simulink model "Mdl_TurnHazard"  (R2024b)
settings: Solver=FixedStepDiscrete  StartTime=0.0  StopTime=10.0  FixedStep=0.1  RelTol=1e-3  EnableMultiTasking=on
values from neighbouring files (symbols this model uses):
  cTH_ONE = mpt.Parameter    [Mdl_TurnHazard_DD.m]
  cTH_THREE = mpt.Parameter    [Mdl_TurnHazard_DD.m]
  cTH_TWO = mpt.Parameter    [Mdl_TurnHazard_DD.m]
undefined symbols (not defined in the file or in its folder): CLUSTER_INACTIVE, eSIGNAL_OK, eTurn_Indicator_ControlIn, tRxSignalId_type_instance, tRxSignalStatus_type_instance, TT_TURN_OFF, TT_TURN_ON, TurnBlink, TurnOff
libraries: simulink x1
settings Model: Creator=aelango6  LastModifiedBy=aelango6
settings DataIOCC: SaveOutput=off
settings OptimizationCC: DefaultParameterBehavior=Inlined  EnhancedBackFolding=on  PassReuseOutputArgsAs=Individual arguments  ZeroExternalMemoryAtStartup=off  ZeroInternalMemoryAtStartup=off  MaxStackSize=750  OptimizeBlockOrder=speed  DifferentSizesBufferReuse=on  OptimizationCustomize=off  EfficientTunableParamExpr=on
settings DebuggingCC: ParameterTunabilityLossMsg=error
settings SFSimCC: MATLABDynamicMemAlloc=off
settings RTWCC: Description=AUTOSAR  SystemTargetFile=autosar.tlc  GenCodeOnly=on  TemplateMakefile=ert_default_tmf  PortableWordSizes=on  DataTypeReplacement=CDataTypesFixedWidth
settings CodeAppCC: ForceParamTrailComments=on  IgnoreCustomStorageClasses=off  OperatorAnnotations=on  SimulinkDataObjDesc=on  SFDataObjDesc=on  InsertBlockDesc=on
settings STFCustomTargetCC: TargetLangStandard=C99 (ISO)  MultiwordLength=256  ParMdlRefBuildCompliant=on  CompOptLevelCompliant=on  IncludeMdlTerminateFcn=off  CombineOutputUpdateFcns=on  SuppressErrorStatus=on  ERTCustomFileBanners=on  SupportNonFinite=off  SupportComplex=off  SupportContinuousTime=off  SupportNonInlinedSFcns=off  RemoveResetFunc=on  ParenthesesLevel=Maximum  CastingMode=Standards  MATLABClassNameForMDSCustomization=Simulink.SoftwareTarget.ERTCustomization  AutosarCompliant=on  UseToolchainInfoCompliant=on  LookupTableObjectStructAxisOrder=2,1,3,4,...  LUTObjectStructOrderEvenSpacing=Size,Table,Breakpoints  SystemTargetFile=autosar.tlc
settings ERTTargetCC: TargetLangStandard=C99 (ISO)  ConcurrentExecutionCompliant=off  IncludeMdlTerminateFcn=off  SuppressErrorStatus=on  SupportNonFinite=off  SupportComplex=off  ParenthesesLevel=Maximum  CastingMode=Standards  ModelStepFunctionPrototypeControlCompliant=off  CPPClassGenCompliant=off  AutosarCompliant=on  LookupTableObjectStructAxisOrder=2,1,3,4,...  LUTObjectStructOrderEvenSpacing=Size,Table,Breakpoints  ERTCustomFileTemplate=example_file_process.tlc  ERTFilePackagingFormat=CompactWithDataFile  BooleanTrueId=TRUE  BooleanFalseId=FALSE

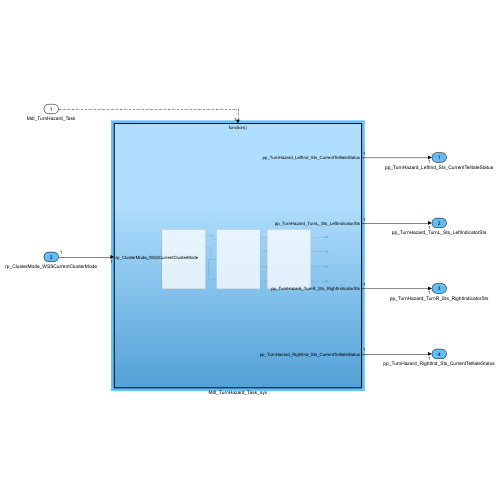
[thumbnail: Simulink's stored preview of the top-level diagram]
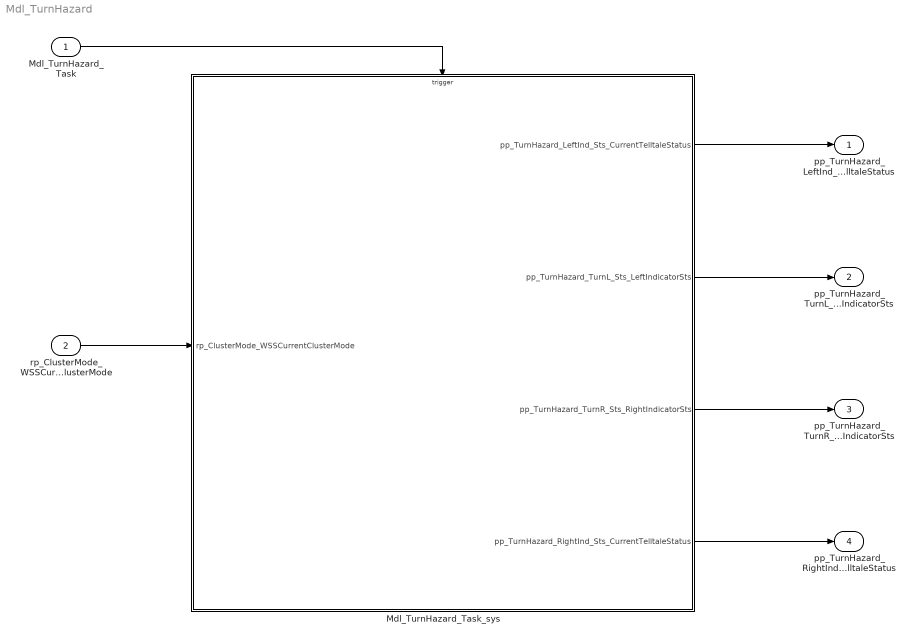
== system Mdl_TurnHazard ==
  Mdl_TurnHazard_Task : Inport  SampleTime=0.1  OutputFunctionCall=on
  rp_ClusterMode_WSSCurrentClusterMode : Inport  Port=2  OutDataTypeStr=ClusterModes  PortDimensions=1
  Mdl_TurnHazard_Task_sys : Subsystem  TreatAsAtomicUnit=on
  pp_TurnHazard_LeftInd_Sts_CurrentTelltaleStatus : Outport  OutDataTypeStr=TT_OP_STATES
  pp_TurnHazard_TurnL_Sts_LeftIndicatorSts : Outport  Port=2  OutDataTypeStr=TurnStates
  pp_TurnHazard_TurnR_Sts_RightIndicatorSts : Outport  Port=3  OutDataTypeStr=TurnStates
  pp_TurnHazard_RightInd_Sts_CurrentTelltaleStatus : Outport  Port=4  OutDataTypeStr=TT_OP_STATES
  wires:
  Mdl_TurnHazard_Task_sys/1(pp_TurnHazard_LeftInd_Sts_CurrentTelltaleStatus) -> pp_TurnHazard_LeftInd_Sts_CurrentTelltaleStatus/1
  Mdl_TurnHazard_Task/1 -> Mdl_TurnHazard_Task_sys/Trigger
  Mdl_TurnHazard_Task_sys/3(pp_TurnHazard_TurnR_Sts_RightIndicatorSts) -> pp_TurnHazard_TurnR_Sts_RightIndicatorSts/1
  rp_ClusterMode_WSSCurrentClusterMode/1 -> Mdl_TurnHazard_Task_sys/1(rp_ClusterMode_WSSCurrentClusterMode)
  Mdl_TurnHazard_Task_sys/2(pp_TurnHazard_TurnL_Sts_LeftIndicatorSts) -> pp_TurnHazard_TurnL_Sts_LeftIndicatorSts/1
  Mdl_TurnHazard_Task_sys/4(pp_TurnHazard_RightInd_Sts_CurrentTelltaleStatus) -> pp_TurnHazard_RightInd_Sts_CurrentTelltaleStatus/1

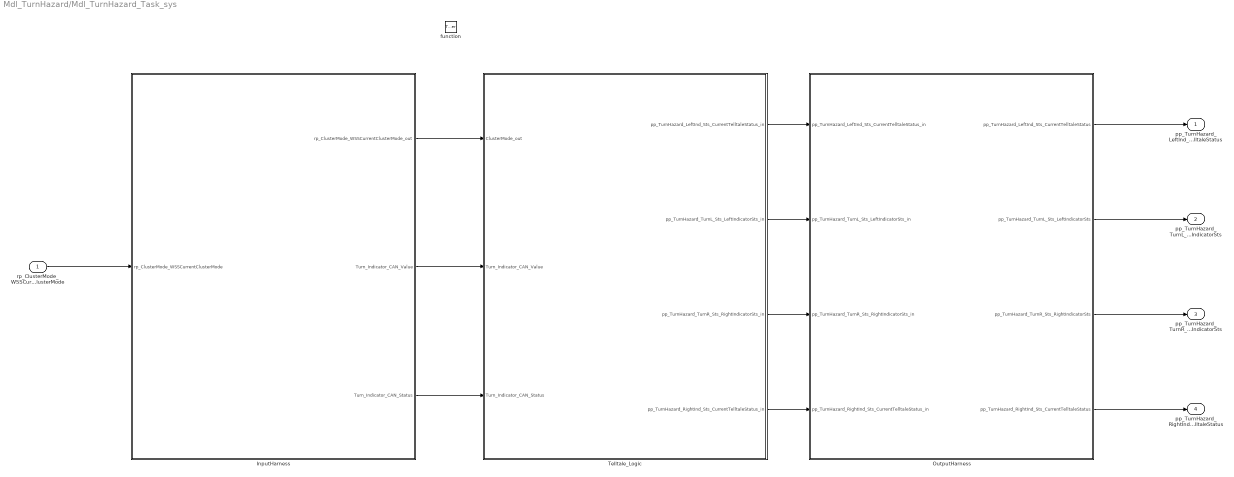
== system Mdl_TurnHazard/Mdl_TurnHazard_Task_sys ==
  rp_ClusterMode_WSSCurrentClusterMode : Inport  OutDataTypeStr=ClusterModes  PortDimensions=1
  function : TriggerPort  TriggerType=function-call  VariantControl=(inherit)  SampleTimeType=periodic  SampleTime=-1
  InputHarness : Subsystem  Variant=on
  OutputHarness : Subsystem  Variant=on
  Telltale_Logic : Subsystem  Description=|
      | Input 1 : Deboune Count
      | Input 2 : Reset Timer Status
      | Output : Timer Debounce Status
  pp_TurnHazard_LeftInd_Sts_CurrentTelltaleStatus : Outport  OutDataTypeStr=TT_OP_STATES  PortDimensions=1
  pp_TurnHazard_TurnL_Sts_LeftIndicatorSts : Outport  Port=2  OutDataTypeStr=TurnStates  PortDimensions=1
  pp_TurnHazard_TurnR_Sts_RightIndicatorSts : Outport  Port=3  OutDataTypeStr=TurnStates  PortDimensions=1
  pp_TurnHazard_RightInd_Sts_CurrentTelltaleStatus : Outport  Port=4  OutDataTypeStr=TT_OP_STATES  PortDimensions=1
  wires:
  rp_ClusterMode_WSSCurrentClusterMode/1 -> InputHarness/1(rp_ClusterMode_WSSCurrentClusterMode)
  InputHarness/1(rp_ClusterMode_WSSCurrentClusterMode_out) -> Telltale_Logic/1(ClusterMode_out)
  InputHarness/3(Turn_Indicator_CAN_Status) -> Telltale_Logic/3(Turn_Indicator_CAN_Status)
  InputHarness/2(Turn_Indicator_CAN_Value) -> Telltale_Logic/2(Turn_Indicator_CAN_Value)
  Telltale_Logic/1(pp_TurnHazard_LeftInd_Sts_CurrentTelltaleStatus_in) -> OutputHarness/1(pp_TurnHazard_LeftInd_Sts_CurrentTelltaleStatus_in)
  Telltale_Logic/2(pp_TurnHazard_TurnL_Sts_LeftIndicatorSts_in) -> OutputHarness/2(pp_TurnHazard_TurnL_Sts_LeftIndicatorSts_in)
  Telltale_Logic/3(pp_TurnHazard_TurnR_Sts_RightIndicatorSts_in) -> OutputHarness/3(pp_TurnHazard_TurnR_Sts_RightIndicatorSts_in)
  Telltale_Logic/4(pp_TurnHazard_RightInd_Sts_CurrentTelltaleStatus_in) -> OutputHarness/4(pp_TurnHazard_RightInd_Sts_CurrentTelltaleStatus_in)
  OutputHarness/1(pp_TurnHazard_LeftInd_Sts_CurrentTelltaleStatus) -> pp_TurnHazard_LeftInd_Sts_CurrentTelltaleStatus/1
  OutputHarness/2(pp_TurnHazard_TurnL_Sts_LeftIndicatorSts) -> pp_TurnHazard_TurnL_Sts_LeftIndicatorSts/1
  OutputHarness/3(pp_TurnHazard_TurnR_Sts_RightIndicatorSts) -> pp_TurnHazard_TurnR_Sts_RightIndicatorSts/1
  OutputHarness/4(pp_TurnHazard_RightInd_Sts_CurrentTelltaleStatus) -> pp_TurnHazard_RightInd_Sts_CurrentTelltaleStatus/1

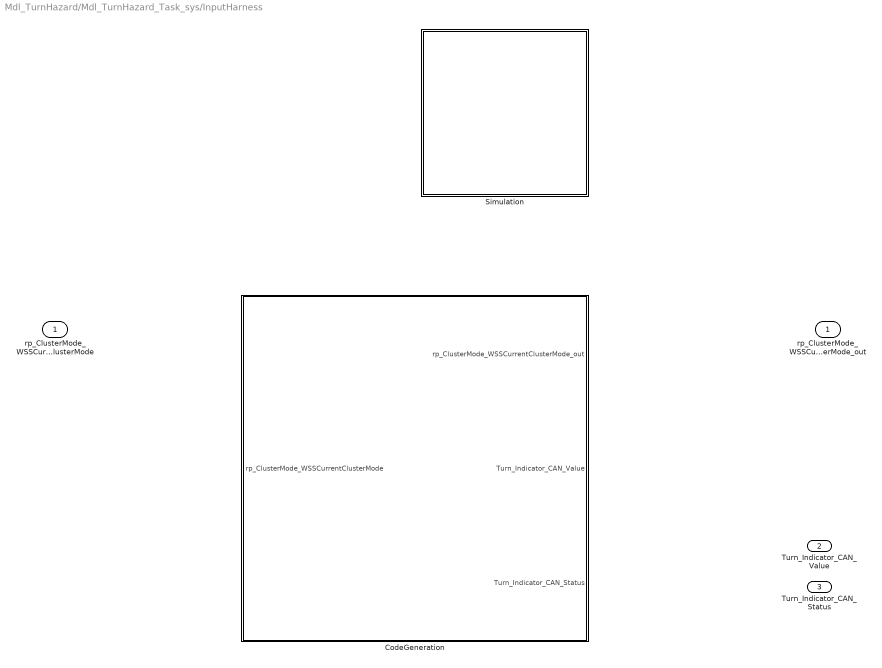
== system Mdl_TurnHazard/Mdl_TurnHazard_Task_sys/InputHarness ==
  rp_ClusterMode_WSSCurrentClusterMode : Inport  OutDataTypeStr=ClusterModes  PortDimensions=1
  CodeGeneration : Subsystem  VariantControl=CODEGENERATION
  Simulation : Subsystem  VariantControl=SIMULATION
  rp_ClusterMode_WSSCurrentClusterMode_out : Outport  OutDataTypeStr=ClusterModes  PortDimensions=1
  Turn_Indicator_CAN_Value : Outport  Port=2
  Turn_Indicator_CAN_Status : Outport  Port=3

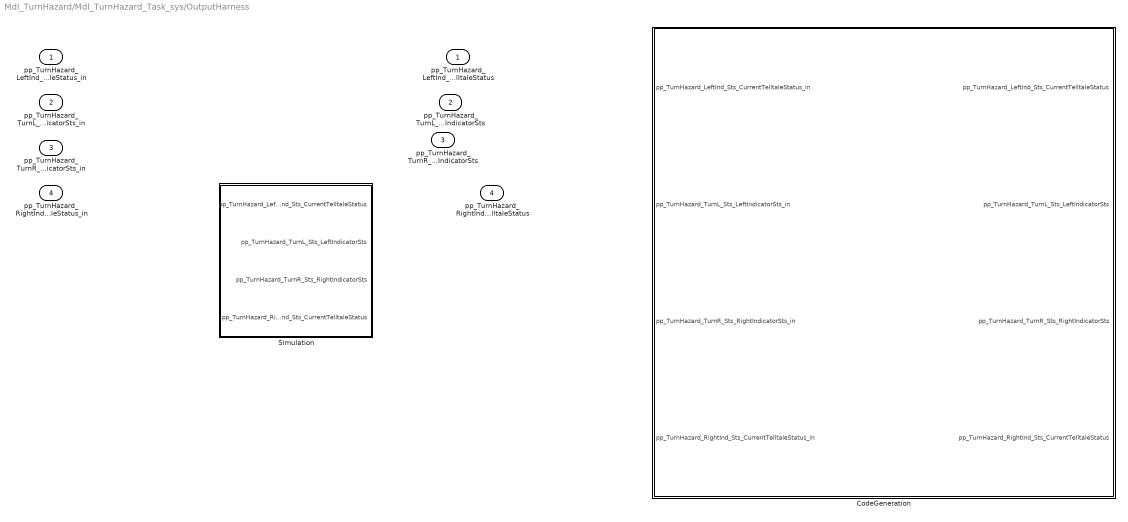
== system Mdl_TurnHazard/Mdl_TurnHazard_Task_sys/OutputHarness ==
  pp_TurnHazard_LeftInd_Sts_CurrentTelltaleStatus_in : Inport  OutDataTypeStr=TT_OP_STATES  PortDimensions=1
  pp_TurnHazard_TurnL_Sts_LeftIndicatorSts_in : Inport  Port=2  OutDataTypeStr=TurnStates  PortDimensions=1
  pp_TurnHazard_TurnR_Sts_RightIndicatorSts_in : Inport  Port=3  OutDataTypeStr=TurnStates  PortDimensions=1
  pp_TurnHazard_RightInd_Sts_CurrentTelltaleStatus_in : Inport  Port=4  OutDataTypeStr=TT_OP_STATES  PortDimensions=1
  CodeGeneration : Subsystem  VariantControl=CODEGENERATION
  Simulation : Subsystem  VariantControl=SIMULATION
  pp_TurnHazard_LeftInd_Sts_CurrentTelltaleStatus : Outport  OutDataTypeStr=TT_OP_STATES  PortDimensions=1
  pp_TurnHazard_TurnL_Sts_LeftIndicatorSts : Outport  Port=2  OutDataTypeStr=TurnStates  PortDimensions=1
  pp_TurnHazard_TurnR_Sts_RightIndicatorSts : Outport  Port=3  OutDataTypeStr=TurnStates  PortDimensions=1
  pp_TurnHazard_RightInd_Sts_CurrentTelltaleStatus : Outport  Port=4  OutDataTypeStr=TT_OP_STATES  PortDimensions=1

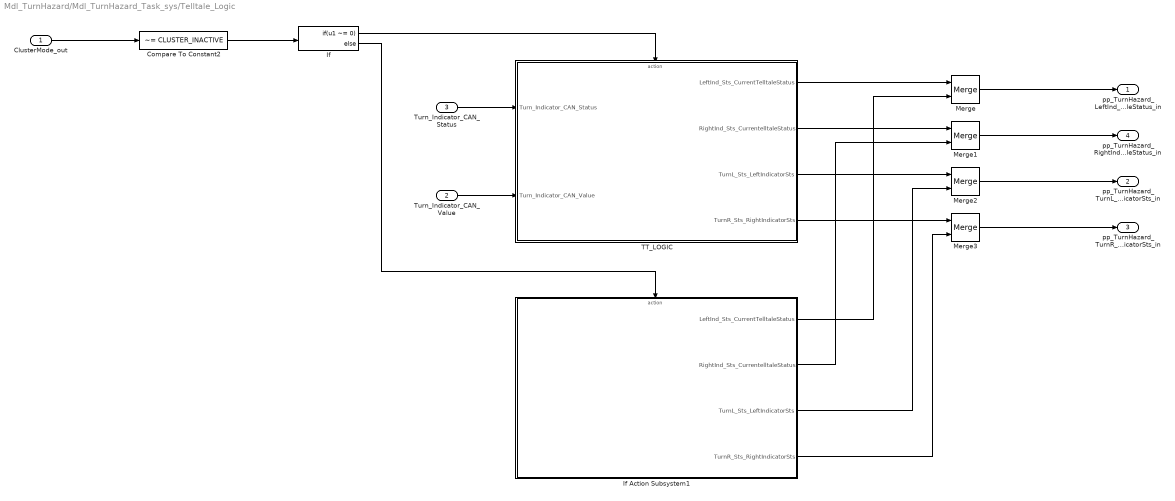
== system Mdl_TurnHazard/Mdl_TurnHazard_Task_sys/Telltale_Logic ==
  ClusterMode_out : Inport  OutDataTypeStr=uint8
  Turn_Indicator_CAN_Value : Inport  Port=2
  Turn_Indicator_CAN_Status : Inport  Port=3
  Compare To Constant2 : simulink/Logic and Bit Operations/Compare To Constant  relop=~=  const=CLUSTER_INACTIVE  OutDataTypeStr=boolean
  If : If  IfExpression=u1 ~= 0
  If Action Subsystem1 : Subsystem  TreatAsAtomicUnit=on
  Merge{,1..3} (4 alike) : Merge
  TT_LOGIC : Subsystem  TreatAsAtomicUnit=on
  pp_TurnHazard_LeftInd_Sts_CurrentTelltaleStatus_in : Outport
  pp_TurnHazard_TurnL_Sts_LeftIndicatorSts_in : Outport  Port=2
  pp_TurnHazard_TurnR_Sts_RightIndicatorSts_in : Outport  Port=3
  pp_TurnHazard_RightInd_Sts_CurrentTelltaleStatus_in : Outport  Port=4
  wires:
  ClusterMode_out/1 -> Compare To Constant2/1
  If/1 -> TT_LOGIC/Action
  If/2 -> If Action Subsystem1/Action
  Compare To Constant2/1 -> If/1
  Turn_Indicator_CAN_Status/1 -> TT_LOGIC/1(Turn_Indicator_CAN_Status)
  Turn_Indicator_CAN_Value/1 -> TT_LOGIC/2(Turn_Indicator_CAN_Value)
  TT_LOGIC/1(LeftInd_Sts_CurrentTelltaleStatus) -> Merge/1
  If Action Subsystem1/1(LeftInd_Sts_CurrentTelltaleStatus) -> Merge/2
  TT_LOGIC/2(RightInd_Sts_CurrentelltaleStatus) -> Merge1/1
  If Action Subsystem1/2(RightInd_Sts_CurrentelltaleStatus) -> Merge1/2
  TT_LOGIC/3(TurnL_Sts_LeftIndicatorSts) -> Merge2/1
  If Action Subsystem1/3(TurnL_Sts_LeftIndicatorSts) -> Merge2/2
  TT_LOGIC/4(TurnR_Sts_RightIndicatorSts) -> Merge3/1
  If Action Subsystem1/4(TurnR_Sts_RightIndicatorSts) -> Merge3/2
  Merge/1 -> pp_TurnHazard_LeftInd_Sts_CurrentTelltaleStatus_in/1
  Merge1/1 -> pp_TurnHazard_RightInd_Sts_CurrentTelltaleStatus_in/1
  Merge2/1 -> pp_TurnHazard_TurnL_Sts_LeftIndicatorSts_in/1
  Merge3/1 -> pp_TurnHazard_TurnR_Sts_RightIndicatorSts_in/1

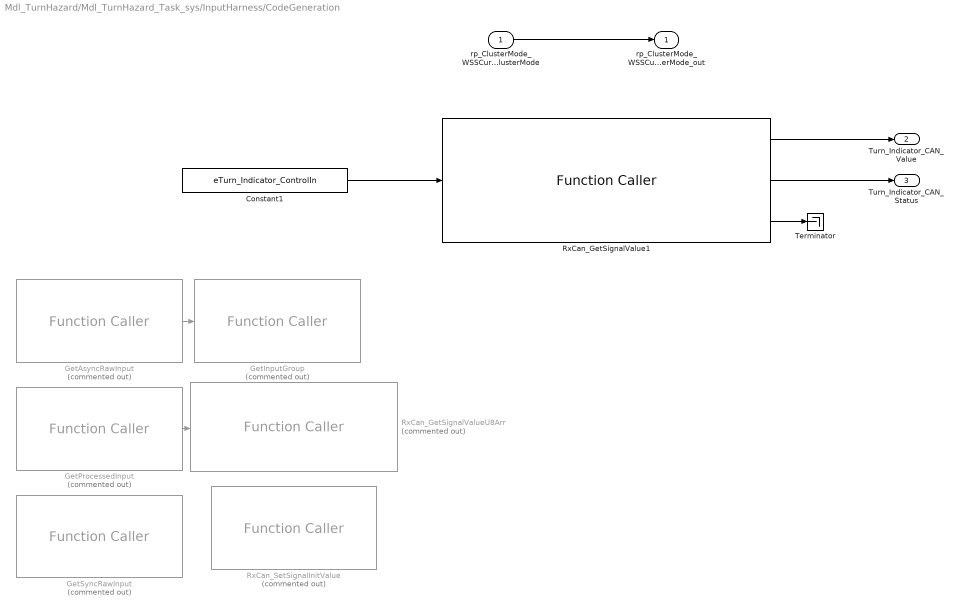
== system Mdl_TurnHazard/Mdl_TurnHazard_Task_sys/InputHarness/CodeGeneration ==
  rp_ClusterMode_WSSCurrentClusterMode : Inport  OutDataTypeStr=ClusterModes  PortDimensions=1
  Constant1 : Constant  Value=eTurn_Indicator_ControlIn
  GetAsyncRawInput : FunctionCaller  Commented=on  FunctionPrototype=[AsyncInput,ErrorStatus,error_status] = GetAsyncRawInput(InputId)  InputArgumentSpecifications=<Enter example>  OutputArgumentSpecifications=<Enter example>
  GetInputGroup : FunctionCaller  Commented=on  FunctionPrototype=[SyncInput,ErrorStatus,error_status] = GetInputGroup(InputId)  InputArgumentSpecifications=<Enter example>  OutputArgumentSpecifications=<Enter example>
  GetProcessedInput : FunctionCaller  Commented=on  FunctionPrototype=[InputSignal,ErrorStatus,error_status] = GetProcessedInput(InputId)  InputArgumentSpecifications=<Enter example>  OutputArgumentSpecifications=<Enter example>
  GetSyncRawInput : FunctionCaller  Commented=on  FunctionPrototype=[SyncInput,ErrorStatus,error_status] = GetSyncRawInput(InputId)  InputArgumentSpecifications=<Enter example>  OutputArgumentSpecifications=<Enter example>
  RxCan_GetSignalValue1 : FunctionCaller  FunctionPrototype=[pSignalValue,pSignalStatus,error_status] = RxCan_GetSignalValue(SignalId)  InputArgumentSpecifications=tRxSignalId_type_instance(1)  OutputArgumentSpecifications=uint8(1) ,tRxSignalStatus_type_instance(1) ,uint8(1)
  RxCan_GetSignalValueU8Arr : FunctionCaller  Commented=on  FunctionPrototype=[pSignalValue,pSignalStatus,pSignalLength,error_status] = RxCan_GetSignalValueU8Arr(SignalId)  InputArgumentSpecifications=<Enter example>  OutputArgumentSpecifications=<Enter example>
  RxCan_SetSignalInitValue : FunctionCaller  Commented=on  FunctionPrototype=[pSignalValue,error_status] = RxCan_SetSignalInitValue(SignalId)  InputArgumentSpecifications=<Enter example>  OutputArgumentSpecifications=<Enter example>
  Terminator : Terminator
  rp_ClusterMode_WSSCurrentClusterMode_out : Outport  OutDataTypeStr=ClusterModes  PortDimensions=1
  Turn_Indicator_CAN_Value : Outport  Port=2
  Turn_Indicator_CAN_Status : Outport  Port=3
  wires:
  rp_ClusterMode_WSSCurrentClusterMode/1 -> rp_ClusterMode_WSSCurrentClusterMode_out/1
  GetProcessedInput/2 -> RxCan_GetSignalValueU8Arr/1
  GetAsyncRawInput/2 -> GetInputGroup/1
  Constant1/1 -> RxCan_GetSignalValue1/1
  RxCan_GetSignalValue1/2 -> Turn_Indicator_CAN_Status/1
  RxCan_GetSignalValue1/1 -> Turn_Indicator_CAN_Value/1
  RxCan_GetSignalValue1/3 -> Terminator/1

== system Mdl_TurnHazard/Mdl_TurnHazard_Task_sys/InputHarness/Simulation ==

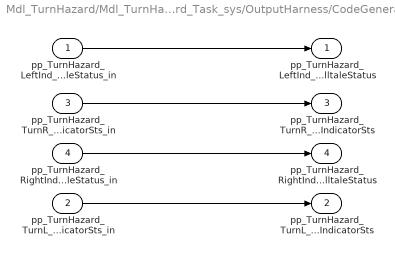
== system Mdl_TurnHazard/Mdl_TurnHazard_Task_sys/OutputHarness/CodeGeneration ==
  pp_TurnHazard_LeftInd_Sts_CurrentTelltaleStatus_in : Inport  OutDataTypeStr=TT_OP_STATES  PortDimensions=1
  pp_TurnHazard_TurnL_Sts_LeftIndicatorSts_in : Inport  Port=2  OutDataTypeStr=TurnStates  PortDimensions=1
  pp_TurnHazard_TurnR_Sts_RightIndicatorSts_in : Inport  Port=3  OutDataTypeStr=TurnStates  PortDimensions=1
  pp_TurnHazard_RightInd_Sts_CurrentTelltaleStatus_in : Inport  Port=4  OutDataTypeStr=TT_OP_STATES  PortDimensions=1
  pp_TurnHazard_LeftInd_Sts_CurrentTelltaleStatus : Outport  OutDataTypeStr=TT_OP_STATES  PortDimensions=1
  pp_TurnHazard_TurnL_Sts_LeftIndicatorSts : Outport  Port=2  OutDataTypeStr=TurnStates  PortDimensions=1
  pp_TurnHazard_TurnR_Sts_RightIndicatorSts : Outport  Port=3  OutDataTypeStr=TurnStates  PortDimensions=1
  pp_TurnHazard_RightInd_Sts_CurrentTelltaleStatus : Outport  Port=4  OutDataTypeStr=TT_OP_STATES  PortDimensions=1
  wires:
  pp_TurnHazard_LeftInd_Sts_CurrentTelltaleStatus_in/1 -> pp_TurnHazard_LeftInd_Sts_CurrentTelltaleStatus/1
  pp_TurnHazard_TurnR_Sts_RightIndicatorSts_in/1 -> pp_TurnHazard_TurnR_Sts_RightIndicatorSts/1
  pp_TurnHazard_RightInd_Sts_CurrentTelltaleStatus_in/1 -> pp_TurnHazard_RightInd_Sts_CurrentTelltaleStatus/1
  pp_TurnHazard_TurnL_Sts_LeftIndicatorSts_in/1 -> pp_TurnHazard_TurnL_Sts_LeftIndicatorSts/1

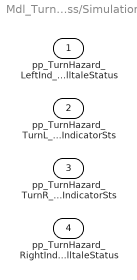
== system Mdl_TurnHazard/Mdl_TurnHazard_Task_sys/OutputHarness/Simulation ==
  pp_TurnHazard_LeftInd_Sts_CurrentTelltaleStatus : Outport  OutDataTypeStr=TT_OP_STATES  PortDimensions=1
  pp_TurnHazard_TurnL_Sts_LeftIndicatorSts : Outport  Port=2  OutDataTypeStr=TurnStates  PortDimensions=1
  pp_TurnHazard_TurnR_Sts_RightIndicatorSts : Outport  Port=3  OutDataTypeStr=TurnStates  PortDimensions=1
  pp_TurnHazard_RightInd_Sts_CurrentTelltaleStatus : Outport  Port=4  OutDataTypeStr=TT_OP_STATES  PortDimensions=1

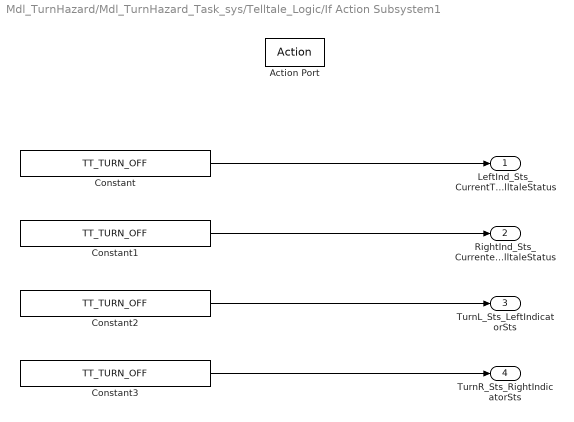
== system Mdl_TurnHazard/Mdl_TurnHazard_Task_sys/Telltale_Logic/If Action Subsystem1 ==
  Action Port : ActionPort  ActionPortLabel=else
  Constant{,1..3} (4 alike) : Constant  Value=TT_TURN_OFF
  LeftInd_Sts_CurrentTelltaleStatus : Outport
  RightInd_Sts_CurrentelltaleStatus : Outport  Port=2
  TurnL_Sts_LeftIndicatorSts : Outport  Port=3
  TurnR_Sts_RightIndicatorSts : Outport  Port=4
  wires:
  Constant/1 -> LeftInd_Sts_CurrentTelltaleStatus/1
  Constant1/1 -> RightInd_Sts_CurrentelltaleStatus/1
  Constant2/1 -> TurnL_Sts_LeftIndicatorSts/1
  Constant3/1 -> TurnR_Sts_RightIndicatorSts/1

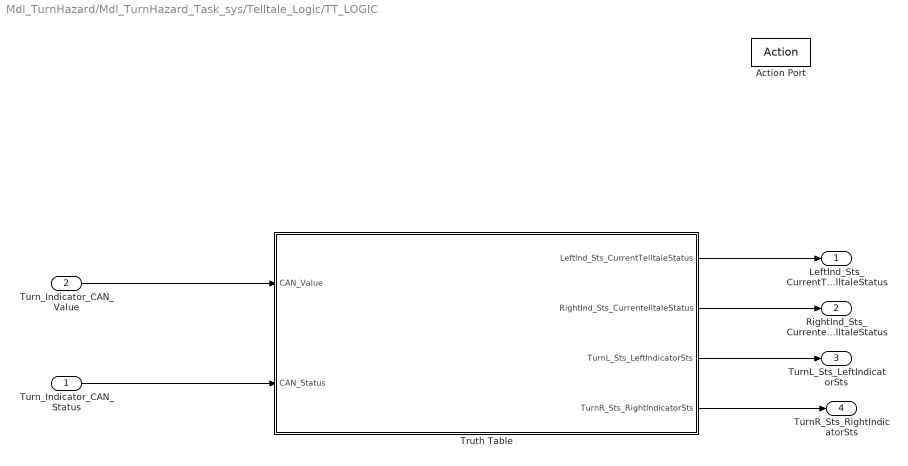
== system Mdl_TurnHazard/Mdl_TurnHazard_Task_sys/Telltale_Logic/TT_LOGIC ==
  Turn_Indicator_CAN_Status : Inport
  Turn_Indicator_CAN_Value : Inport  Port=2
  Action Port : ActionPort  ActionPortLabel=if(u1 ~= 0)
  Truth Table : Truth Table  TreatAsAtomicUnit=on
  LeftInd_Sts_CurrentTelltaleStatus : Outport
  RightInd_Sts_CurrentelltaleStatus : Outport  Port=2
  TurnL_Sts_LeftIndicatorSts : Outport  Port=3
  TurnR_Sts_RightIndicatorSts : Outport  Port=4
  wires:
  Turn_Indicator_CAN_Status/1 -> Truth Table/2(CAN_Status)
  Turn_Indicator_CAN_Value/1 -> Truth Table/1(CAN_Value)
  Truth Table/1(LeftInd_Sts_CurrentTelltaleStatus) -> LeftInd_Sts_CurrentTelltaleStatus/1
  Truth Table/2(RightInd_Sts_CurrentelltaleStatus) -> RightInd_Sts_CurrentelltaleStatus/1
  Truth Table/4(TurnR_Sts_RightIndicatorSts) -> TurnR_Sts_RightIndicatorSts/1
  Truth Table/3(TurnL_Sts_LeftIndicatorSts) -> TurnL_Sts_LeftIndicatorSts/1

== matlab function Mdl_TurnHazard/Mdl_TurnHazard_Task_sys/Telltale_Logic/TT_LOGIC/Truth Table ==
  data: CAN_Value input; LeftInd_Sts_CurrentTelltaleStatus output; RightInd_Sts_CurrentelltaleStatus output; TurnL_Sts_LeftIndicatorSts output; CAN_Status input; TurnR_Sts_RightIndicatorSts output; TT_TURN_OFF parameter; TT_TURN_ON parameter; eSIGNAL_OK parameter; TurnOff parameter; cTH_ONE parameter; cTH_TWO parameter; cTH_THREE parameter; TurnBlink parameter double
function [LeftInd_Sts_CurrentTelltaleStatus, RightInd_Sts_CurrentelltaleStatus, TurnL_Sts_LeftIndicatorSts, TurnR_Sts_RightIndicatorSts] = fcn(CAN_Value, CAN_Status, TT_TURN_OFF, TT_TURN_ON, eSIGNAL_OK, TurnOff, cTH_ONE, cTH_TWO, cTH_THREE, TurnBlink)

aVarTruthTableCondition_1 = false;
aVarTruthTableCondition_2 = false;
aVarTruthTableCondition_3 = false;
aVarTruthTableCondition_4 = false;


% TT_Left = Off
% TT_Right = Off

aVarTruthTableCondition_1 = logical((CAN_Status ~= eSIGNAL_OK) || (CAN_Value == TurnOff));

% TT_Left = On

aVarTruthTableCondition_2 = logical(CAN_Value == cTH_ONE);

% TT_Right = On

aVarTruthTableCondition_3 = logical(CAN_Value == cTH_TWO);

% Both TT Blink - Hazard

aVarTruthTableCondition_4 = logical(CAN_Value == cTH_THREE);

if (aVarTruthTableCondition_1)
    aFcnTruthTableAction_1();
elseif (aVarTruthTableCondition_2)
    aFcnTruthTableAction_2();
elseif (aVarTruthTableCondition_3)
    aFcnTruthTableAction_3();
elseif (aVarTruthTableCondition_4)
    aFcnTruthTableAction_4();
else % Default
    aFcnTruthTableAction_1();
end

function aFcnTruthTableAction_1()

% Left and Right Telltales are off

RightInd_Sts_CurrentelltaleStatus=TT_TURN_OFF;
LeftInd_Sts_CurrentTelltaleStatus = TT_TURN_OFF;
TurnR_Sts_RightIndicatorSts = TT_TURN_OFF;
TurnL_Sts_LeftIndicatorSts = TT_TURN_OFF;

function aFcnTruthTableAction_2()

% TT_Left = On

RightInd_Sts_CurrentelltaleStatus=TT_TURN_OFF;
LeftInd_Sts_CurrentTelltaleStatus = TT_TURN_ON;
TurnR_Sts_RightIndicatorSts = TT_TURN_OFF;
TurnL_Sts_LeftIndicatorSts = TT_TURN_ON;

function aFcnTruthTableAction_3()

% TT_Right = On

RightInd_Sts_CurrentelltaleStatus=TT_TURN_ON;
LeftInd_Sts_CurrentTelltaleStatus = TT_TURN_OFF;
TurnR_Sts_RightIndicatorSts = TT_TURN_ON;
TurnL_Sts_LeftIndicatorSts = TT_TURN_OFF;

function aFcnTruthTableAction_4()

% Both TT Blink - Hazard

RightInd_Sts_CurrentelltaleStatus=TurnBlink;
LeftInd_Sts_CurrentTelltaleStatus = TurnBlink;
TurnR_Sts_RightIndicatorSts = TurnBlink;
TurnL_Sts_LeftIndicatorSts = TurnBlink;
